simulink model "roll_sim"  (R2018b)
settings: Solver=VariableStepAuto  StartTime=0.0  StopTime=10.0  RelTol=1e-3
settings Model: Creator=a4327  LastModifiedBy=a4327

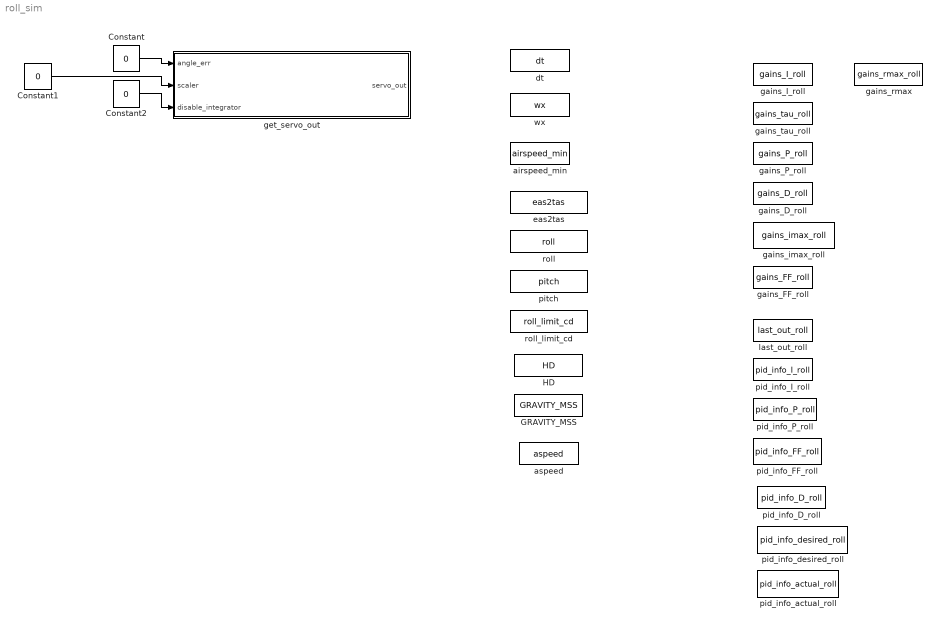
== system roll_sim ==
  Constant : Constant  Value=0
  Constant1 : Constant  Value=0
  Constant2 : Constant  Value=0
  GRAVITY_MSS : DataStoreMemory  DataStoreName=GRAVITY_MSS  ReadBeforeWriteMsg=warning  WriteAfterWriteMsg=warning  WriteAfterReadMsg=warning  InitialValue=GRAVITY_MSS  ShowAdditionalParam=off  OutDataTypeStr=double
  HD : DataStoreMemory  DataStoreName=HD  ReadBeforeWriteMsg=warning  WriteAfterWriteMsg=warning  WriteAfterReadMsg=warning  InitialValue=HD  ShowAdditionalParam=off  OutDataTypeStr=double
  airspeed_min : DataStoreMemory  DataStoreName=airspeed_min  ReadBeforeWriteMsg=warning  WriteAfterWriteMsg=warning  WriteAfterReadMsg=warning  InitialValue=airspeed_min  ShowAdditionalParam=off  OutDataTypeStr=double
  aspeed : DataStoreMemory  DataStoreName=aspeed  ReadBeforeWriteMsg=warning  WriteAfterWriteMsg=warning  WriteAfterReadMsg=warning  InitialValue=aspeed  ShowAdditionalParam=off  OutDataTypeStr=double
  dt : DataStoreMemory  DataStoreName=dt  ReadBeforeWriteMsg=warning  WriteAfterWriteMsg=warning  WriteAfterReadMsg=warning  InitialValue=dt  ShowAdditionalParam=off  OutDataTypeStr=double
  eas2tas : DataStoreMemory  DataStoreName=eas2tas  ReadBeforeWriteMsg=warning  WriteAfterWriteMsg=warning  WriteAfterReadMsg=warning  InitialValue=eas2tas  ShowAdditionalParam=off  OutDataTypeStr=double
  gains_D_roll : DataStoreMemory  DataStoreName=gains_D_roll  ReadBeforeWriteMsg=warning  WriteAfterWriteMsg=warning  WriteAfterReadMsg=warning  InitialValue=gains_D_roll  ShowAdditionalParam=off  OutDataTypeStr=double
  gains_FF_roll : DataStoreMemory  DataStoreName=gains_FF_roll  ReadBeforeWriteMsg=warning  WriteAfterWriteMsg=warning  WriteAfterReadMsg=warning  InitialValue=gains_FF_roll  ShowAdditionalParam=off  OutDataTypeStr=double
  gains_I_roll : DataStoreMemory  DataStoreName=gains_I_roll  ReadBeforeWriteMsg=warning  WriteAfterWriteMsg=warning  WriteAfterReadMsg=warning  InitialValue=gains_I_roll  ShowAdditionalParam=off  OutDataTypeStr=double
  gains_P_roll : DataStoreMemory  DataStoreName=gains_P_roll  ReadBeforeWriteMsg=warning  WriteAfterWriteMsg=warning  WriteAfterReadMsg=warning  InitialValue=gains_P_roll  ShowAdditionalParam=off  OutDataTypeStr=double
  gains_imax_roll : DataStoreMemory  DataStoreName=gains_imax_roll  ReadBeforeWriteMsg=warning  WriteAfterWriteMsg=warning  WriteAfterReadMsg=warning  InitialValue=gains_imax_roll  ShowAdditionalParam=off  OutDataTypeStr=double
  gains_rmax : DataStoreMemory  DataStoreName=gains_rmax_roll  ReadBeforeWriteMsg=warning  WriteAfterWriteMsg=warning  WriteAfterReadMsg=warning  InitialValue=gains_rmax_roll  ShowAdditionalParam=off  OutDataTypeStr=double
  gains_tau_roll : DataStoreMemory  DataStoreName=gains_tau_roll  ReadBeforeWriteMsg=warning  WriteAfterWriteMsg=warning  WriteAfterReadMsg=warning  InitialValue=gains_tau_roll  ShowAdditionalParam=off  OutDataTypeStr=double
  get_servo_out : MATLAB Function  TreatAsAtomicUnit=on
  last_out_roll : DataStoreMemory  DataStoreName=last_out_roll  ReadBeforeWriteMsg=warning  WriteAfterWriteMsg=warning  WriteAfterReadMsg=warning  InitialValue=last_out_roll  ShowAdditionalParam=off  OutDataTypeStr=double
  pid_info_D_roll : DataStoreMemory  DataStoreName=pid_info_D_roll  ReadBeforeWriteMsg=warning  WriteAfterWriteMsg=warning  WriteAfterReadMsg=warning  InitialValue=pid_info_D_roll  ShowAdditionalParam=off  OutDataTypeStr=double
  pid_info_FF_roll : DataStoreMemory  DataStoreName=pid_info_FF_roll  ReadBeforeWriteMsg=warning  WriteAfterWriteMsg=warning  WriteAfterReadMsg=warning  InitialValue=pid_info_FF_roll  ShowAdditionalParam=off  OutDataTypeStr=double
  pid_info_I_roll : DataStoreMemory  DataStoreName=pid_info_I_roll  ReadBeforeWriteMsg=warning  WriteAfterWriteMsg=warning  WriteAfterReadMsg=warning  InitialValue=pid_info_I_roll  ShowAdditionalParam=off  OutDataTypeStr=double
  pid_info_P_roll : DataStoreMemory  DataStoreName=pid_info_P_roll  ReadBeforeWriteMsg=warning  WriteAfterWriteMsg=warning  WriteAfterReadMsg=warning  InitialValue=pid_info_P_roll  ShowAdditionalParam=off  OutDataTypeStr=double
  pid_info_actual_roll : DataStoreMemory  DataStoreName=pid_info_actual_roll  ReadBeforeWriteMsg=warning  WriteAfterWriteMsg=warning  WriteAfterReadMsg=warning  InitialValue=pid_info_actual_roll  ShowAdditionalParam=off  OutDataTypeStr=double
  pid_info_desired_roll : DataStoreMemory  DataStoreName=pid_info_desired_roll  ReadBeforeWriteMsg=warning  WriteAfterWriteMsg=warning  WriteAfterReadMsg=warning  InitialValue=pid_info_desired_roll  ShowAdditionalParam=off  OutDataTypeStr=double
  pitch : DataStoreMemory  DataStoreName=pitch  ReadBeforeWriteMsg=warning  WriteAfterWriteMsg=warning  WriteAfterReadMsg=warning  InitialValue=pitch  ShowAdditionalParam=off  OutDataTypeStr=double
  roll : DataStoreMemory  DataStoreName=roll  ReadBeforeWriteMsg=warning  WriteAfterWriteMsg=warning  WriteAfterReadMsg=warning  InitialValue=roll  ShowAdditionalParam=off  OutDataTypeStr=double
  roll_limit_cd : DataStoreMemory  DataStoreName=roll_limit_cd  ReadBeforeWriteMsg=warning  WriteAfterWriteMsg=warning  WriteAfterReadMsg=warning  InitialValue=roll_limit_cd  ShowAdditionalParam=off  OutDataTypeStr=double
  wx : DataStoreMemory  DataStoreName=wx  ReadBeforeWriteMsg=warning  WriteAfterWriteMsg=warning  WriteAfterReadMsg=warning  InitialValue=wx  ShowAdditionalParam=off  OutDataTypeStr=double
  wires:
  Constant/1 -> get_servo_out/1(angle_err)
  Constant1/1 -> get_servo_out/2(scaler)
  Constant2/1 -> get_servo_out/3(disable_integrator)

== matlab function roll_sim/get_servo_out ==
  data: angle_err input; servo_out output; scaler input; disable_integrator input; dt data_store_memory; gains_I_roll data_store_memory; gains_tau_roll data_store_memory; gains_P_roll data_store_memory; gains_D_roll data_store_memory; gains_imax_roll data_store_memory; gains_FF_roll data_store_memory; airspeed_min data_store_memory; last_out_roll data_store_memory; pid_info_I_roll data_store_memory; pid_info_P_roll data_store_memory; pid_info_FF_roll data_store_memory; pid_info_D_roll data_store_memory; pid_info_desired_roll data_store_memory; pid_info_actual_roll data_store_memory; eas2tas data_store_memory; roll data_store_memory; pitch data_store_memory; roll_limit_cd data_store_memory; aspeed data_store_memory; gains_rmax_roll data_store_memory; GRAVITY_MSS data_store_memory; wx data_store_memory; HD data_store_memory
function servo_out=get_servo_out(  angle_err,   scaler,   disable_integrator)

servo_out=get_servo_out_roll(  angle_err,   scaler,   disable_integrator);
